simulink model "simulation"  (R2020b)
settings: Solver=VariableStepAuto  StartTime=0.0  StopTime=40  FixedStep=1e-3  RelTol=1e-3
values from neighbouring files (symbols this model uses):
  A0 = A- k*e1'    [script.m]
  ap = ssp.A'    [script.m]
  bp = ssp.C'    [script.m]
  c1 = 1    [script.m]
  c2 = 1    [script.m]
  cp = ssp.B'    [script.m]
  d1 = 1    [script.m]
  d2 = 1    [script.m]
  dp = 0    [script.m]
  e2 = [0 1]'    [script.m]
  gamma = 1    [script.m]
  Gamma = eye(3)    [script.m]
  k = 10*ones(n, 1)    [script.m]
  kp = 1    [script.m]
  rho0 = 0    [script.m]
  theta0 = zeros(3 , 1)    [script.m]
  x0p = zeros(n, 1)    [script.m]
settings Model: Creator=lucas  LastModifiedBy=lucas

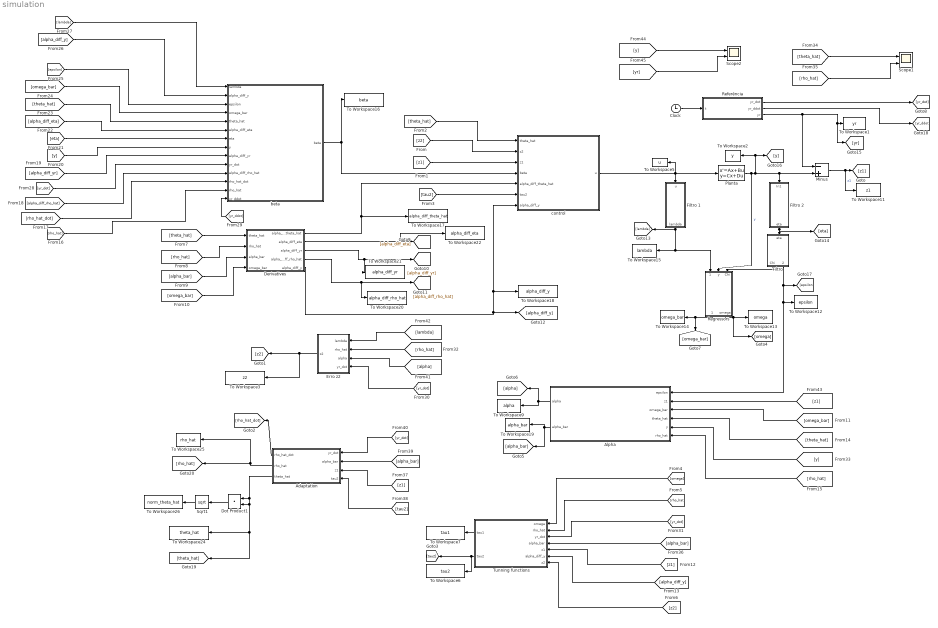
== system simulation ==
  Adaptation : Subsystem
  Alpha : MATLAB Function  TreatAsAtomicUnit=on
  Clock : Clock
  Derivatives : MATLAB Function  TreatAsAtomicUnit=on
  Dot Product1 : DotProduct  InputSameDT=on  OutDataTypeStr=Inherit: Inherit via internal rule
  Erro z2 : MATLAB Function  TreatAsAtomicUnit=on
  Filtro : MATLAB Function  TreatAsAtomicUnit=on
  Filtro 1 : Subsystem
  Filtro 2 : Subsystem
  Minus : Sum  Inputs=-+
  Planta : StateSpace  A=ap  B=bp  C=cp  D=dp  InitialCondition=x0p
  Referência : MATLAB Function  TreatAsAtomicUnit=on
  Regressors : MATLAB Function  TreatAsAtomicUnit=on
  Scope1 : Scope  NumInputPorts=2
  Scope2 : Scope  NumInputPorts=2
  Sqrt1 : Sqrt  SaturateOnIntegerOverflow=on
  To Workspace1 : ToWorkspace  VariableName=yr  SaveFormat=Timeseries  SampleTime=-1
  To Workspace11 : ToWorkspace  VariableName=z1  SaveFormat=Timeseries  SampleTime=-1
  To Workspace12 : ToWorkspace  VariableName=epsilon  SaveFormat=Timeseries  SampleTime=-1
  To Workspace13 : ToWorkspace  VariableName=omega  SaveFormat=Timeseries  SampleTime=-1
  To Workspace14 : ToWorkspace  VariableName=omega_bar  SaveFormat=Timeseries  SampleTime=-1
  To Workspace15 : ToWorkspace  VariableName=lambda  SaveFormat=Timeseries  SampleTime=-1
  To Workspace16 : ToWorkspace  VariableName=beta  SaveFormat=Timeseries  SampleTime=-1
  To Workspace17 : ToWorkspace  VariableName=alpha_diff_theta_hat  SaveFormat=Timeseries  SampleTime=-1
  To Workspace18 : ToWorkspace  VariableName=alpha_diff_y  SaveFormat=Timeseries  SampleTime=-1
  To Workspace19 : ToWorkspace  VariableName=alpha_bar  SaveFormat=Timeseries  SampleTime=-1
  To Workspace2 : ToWorkspace  VariableName=y  SaveFormat=Timeseries  SampleTime=-1
  To Workspace20 : ToWorkspace  VariableName=alpha_diff_rho_hat  SaveFormat=Timeseries  SampleTime=-1
  To Workspace21 : ToWorkspace  VariableName=alpha_diff_yr  SaveFormat=Timeseries  SampleTime=-1
  To Workspace22 : ToWorkspace  VariableName=alpha_diff_eta  SaveFormat=Timeseries  SampleTime=-1
  To Workspace24 : ToWorkspace  VariableName=theta_hat  SaveFormat=Timeseries  SampleTime=-1
  To Workspace25 : ToWorkspace  VariableName=rho_hat  SaveFormat=Timeseries  SampleTime=-1
  To Workspace26 : ToWorkspace  VariableName=norm_theta_hat  SaveFormat=Timeseries  SampleTime=-1
  To Workspace3 : ToWorkspace  VariableName=z2  SaveFormat=Timeseries  SampleTime=-1
  To Workspace5 : ToWorkspace  VariableName=u  SaveFormat=Timeseries  SampleTime=-1
  To Workspace6 : ToWorkspace  VariableName=tau2  SaveFormat=Timeseries  SampleTime=-1
  To Workspace7 : ToWorkspace  VariableName=tau1  SaveFormat=Timeseries  SampleTime=-1
  To Workspace9 : ToWorkspace  VariableName=alpha  SaveFormat=Timeseries  SampleTime=-1
  Tunning functions : MATLAB Function  TreatAsAtomicUnit=on
  beta : MATLAB Function  TreatAsAtomicUnit=on
  control : MATLAB Function  TreatAsAtomicUnit=on
  wires:
  [yr] -> Scope2/2
  [y] -> Scope2/1
  [alpha] -> Erro z2/3(alpha)
  Dot Product1/1 -> Sqrt1/1
  Sqrt1/1 -> To Workspace26/1
  [y] -> Alpha/5(y)
  Alpha/1(alpha) -> [alpha], To Workspace9/1
  [theta_hat] -> Alpha/4(theta_hat)
  [rho_hat] -> Alpha/6(rho_hat)
  Alpha/2(alpha_bar) -> To Workspace19/1, [alpha_bar]
  [z1] -> Alpha/2(z1)
  [omega_bar] -> beta/4(omega_bar)
  Derivatives/5(alpha_diff_y) -> control/7(alpha_diff_y), To Workspace18/1, [alpha_diff_y]
  Derivatives/1(alpha_diff_theta_hat) -> control/5(alpha_diff_theta_hat), To Workspace17/1
  [alpha_diff_y] -> beta/2(alpha_diff_y)
  [rho_hat] -> beta/13(rho_hat)
  [epsilon] -> beta/3(epsilon)
  [z2] -> control/2(z2)
  [lambda] -> beta/1(lambda)
  [alpha_diff_y] -> Tunning functions/6(alpha_diff_y)
  [theta_hat] -> beta/5(theta_hat)
  [eta] -> beta/7(eta)
  [omega_bar] -> Derivatives/4(omega_bar)
  [alpha_diff_yr] -> beta/9(alpha_diff_yr)
  [rho_hat] -> Tunning functions/2(rho_hat)
  [alpha_bar] -> Derivatives/3(alpha_bar)
  beta/1(beta) -> To Workspace16/1, control/4(beta)
  Derivatives/2(alpha_diff_eta) -> To Workspace22/1, [alpha_diff_eta]
  Regressors/1(omega_bar) -> To Workspace14/1, [omega_bar]
  Derivatives/4(alpha_diff_rho_hat) -> To Workspace20/1, [alpha_diff_rho_hat]
  Tunning functions/2(tau2) -> [tau2], To Workspace6/1
  [tau2] -> control/6(tau2)
  control/1(u) -> Filtro 1/1(u), To Workspace5/1, Planta/1
  [z1] -> control/3(z1)
  Filtro 1/1(lambda) -> Regressors/1(lambda), To Workspace15/1, [lambda]
  Planta/1 -> Minus/2, Filtro 2/1(In1), [y], To Workspace2/1, Regressors/2(y)  "y"
  Filtro 2/1(eta) -> Filtro/1(eta), [eta]
  Filtro/2(epsilon) -> Alpha/1(epsilon), To Workspace12/1, [epsilon]
  [alpha_diff_eta] -> beta/6(alpha_diff_eta)
  Referência/1(yr_dot) -> [yr_dot]
  [y] -> beta/8(y)
  [alpha_diff_rho_hat] -> beta/11(alpha_diff_rho_hat)
  Clock/1 -> Referência/1(t)
  Referência/2(yr_ddot) -> [yr_ddot]
  [theta_hat] -> Derivatives/1(theta_hat)
  Derivatives/3(alpha_diff_yr) -> To Workspace21/1, [alpha_diff_yr]
  [rho_hat_dot] -> beta/12(rho_hat_dot)
  [yr_ddot] -> beta/14(yr_ddot)
  [z2] -> Tunning functions/7(z2)
  [yr_dot] -> beta/10(yr_dot)
  [z1] -> Tunning functions/5(z1)
  [theta_hat] -> Scope1/1
  Tunning functions/1(tau1) -> To Workspace7/1
  [alpha_bar] -> Tunning functions/4(alpha_bar)
  [rho_hat] -> Scope1/2
  [rho_hat] -> Erro z2/2(rho_hat)
  Referência/3(yr) -> Minus/1, [yr], To Workspace1/1
  [omega_bar] -> Alpha/3(omega_bar)
  [rho_hat] -> Derivatives/2(rho_hat)
  [yr_dot] -> Erro z2/4(yr_dot)
  Minus/1 -> To Workspace11/1, [z1]  "z1"
  [lambda] -> Erro z2/1(lambda)
  [alpha_bar] -> Adaptation/2(alpha_bar)
  Adaptation/1(rho_hat_dot) -> [rho_hat_dot]
  [theta_hat] -> control/1(theta_hat)
  Adaptation/2(rho_hat) -> To Workspace25/1, [rho_hat]
  [omega] -> Tunning functions/1(omega)
  [yr_dot] -> Adaptation/1(yr_dot)
  [z1] -> Adaptation/3(z1)
  [yr_dot] -> Tunning functions/3(yr_dot)
  Adaptation/3(theta_hat) -> [theta_hat], To Workspace24/1, Dot Product1/2, Dot Product1/1
  [tau2] -> Adaptation/4(tau2)
  Regressors/2(omega) -> To Workspace13/1, [omega]
  Erro z2/1(z2) -> To Workspace3/1, [z2]
  Filtro/1(Chi) -> Regressors/3(Chi)

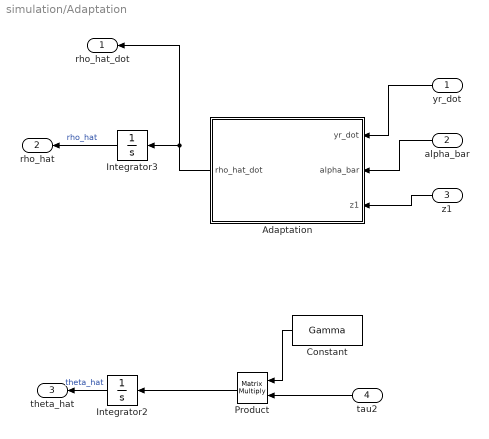
== system simulation/Adaptation ==
  yr_dot : Inport
  alpha_bar : Inport  Port=2
  z1 : Inport  Port=3
  tau2 : Inport  Port=4
  Adaptation : MATLAB Function  TreatAsAtomicUnit=on
  Constant : Constant  Value=Gamma  VectorParams1D=off
  Integrator2 : Integrator  InitialCondition=theta0
  Integrator3 : Integrator  InitialCondition=rho0
  Product : Product  Multiplication=Matrix(*)
  rho_hat_dot : Outport
  rho_hat : Outport  Port=2
  theta_hat : Outport  Port=3
  wires:
  Adaptation/1(rho_hat_dot) -> rho_hat_dot/1, Integrator3/1
  z1/1 -> Adaptation/3(z1)
  tau2/1 -> Product/2
  yr_dot/1 -> Adaptation/1(yr_dot)
  Constant/1 -> Product/1
  Product/1 -> Integrator2/1
  Integrator3/1 -> rho_hat/1  "rho_hat"
  alpha_bar/1 -> Adaptation/2(alpha_bar)
  Integrator2/1 -> theta_hat/1  "theta_hat"

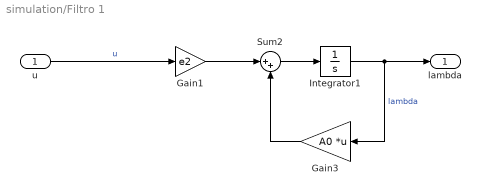
== system simulation/Filtro 1 ==
  u : Inport
  Gain1 : Gain  Gain=e2
  Gain3 : Gain  Gain=A0  Multiplication=Matrix(K*u) (u vector)
  Integrator1 : Integrator
  Sum2 : Sum  Inputs=|++
  lambda : Outport
  wires:
  u/1 -> Gain1/1  "u"
  Sum2/1 -> Integrator1/1
  Gain3/1 -> Sum2/2
  Gain1/1 -> Sum2/1
  Integrator1/1 -> lambda/1, Gain3/1  "lambda"

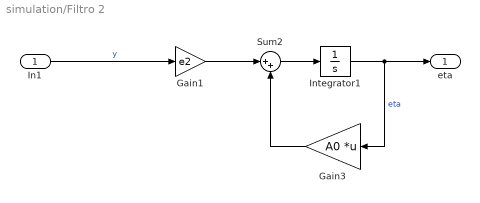
== system simulation/Filtro 2 ==
  In1 : Inport
  Gain1 : Gain  Gain=e2
  Gain3 : Gain  Gain=A0  Multiplication=Matrix(K*u) (u vector)
  Integrator1 : Integrator
  Sum2 : Sum  Inputs=|++
  eta : Outport
  wires:
  In1/1 -> Gain1/1  "y"
  Sum2/1 -> Integrator1/1
  Gain3/1 -> Sum2/2
  Gain1/1 -> Sum2/1
  Integrator1/1 -> eta/1, Gain3/1  "eta"

== matlab function simulation/control ==
  data: theta_hat input; u output; z2 input; z1 input; beta input; alpha_diff_theta_hat input; tau2 input; alpha_diff_y input; c2 parameter; d2 parameter; Gamma parameter
function u = control(theta_hat, z2, z1, beta, alpha_diff_theta_hat, tau2, alpha_diff_y, c2, d2, Gamma)
    kp_hat = theta_hat(1);
    u = -c2*z2;
    u = u - kp_hat*z1;
    u = u + beta;
    u = u + alpha_diff_theta_hat*Gamma*tau2;
    u = u - d2*(alpha_diff_y^2)*z2;

== matlab function simulation/Tunning functions ==
  data: omega input; tau1 output; rho_hat input; yr_dot input; alpha_bar input; z1 input; tau2 output; alpha_diff_y input; z2 input; e1_tau parameter
function [tau1, tau2] = tunning(omega, rho_hat, yr_dot, alpha_bar, z1, alpha_diff_y, z2, e1_tau)
    omega_0 = omega-(rho_hat*(yr_dot+alpha_bar)*e1_tau);
    tau1 = omega_0*z1;
    tau2 = tau1 - (alpha_diff_y*omega*z2);

== matlab function simulation/Referência ==
  data: yr_dot output; yr_ddot output; t input; yr output
function [yr_dot, yr_ddot, yr] = reference(t)
    yr = 2 + 5*sin(t) + 5*sin(3.7*t);
    yr_dot = 5*cos(t) + 5*3.7*cos(3.7*t);
    yr_ddot = -5*sin(t) - 5*3.7*3.7*sin(3.7*t);

== matlab function simulation/Erro z2 ==
  data: lambda input; z2 output; rho_hat input; alpha input; yr_dot input
function z2 = erro(lambda, rho_hat, alpha, yr_dot)
    z2 = lambda(2)-rho_hat*yr_dot - alpha;

== matlab function simulation/Adaptation/Adaptation ==
  data: yr_dot input; rho_hat_dot output; alpha_bar input; z1 input; gamma parameter; kp parameter
function rho_hat_dot  = adaptation(yr_dot, alpha_bar, z1, gamma, kp)
    rho_hat_dot = -gamma*sign(kp)*(yr_dot+alpha_bar)*z1;

== matlab function simulation/Alpha ==
  data: epsilon input; alpha output; z1 input; omega_bar input; theta_hat input; y input; rho_hat input; alpha_bar output; c1 parameter; d1 parameter
function [alpha, alpha_bar] = alpha(epsilon,z1, omega_bar, theta_hat, y, rho_hat, c1, d1)
    alpha_bar = -(c1*z1)-(d1*z1)-epsilon(2)-(dot(omega_bar, theta_hat));
    alpha = rho_hat*alpha_bar;

== matlab function simulation/Filtro ==
  data: Chi output; eta input; epsilon output; A0 parameter
function [Chi, epsilon] = filtro(eta, A0)
    Chi = -[A0*eta eta];
    epsilon = -A0*A0*eta;

== matlab function simulation/Regressors ==
  data: lambda input; y input; omega_bar output; omega output; Chi input; e1 parameter
function [omega_bar, omega] = fcn(lambda, y, Chi, e1)
aux = Chi(2,:) - y*e1';
omega_bar = [0 aux]';
omega = [lambda(2) aux]';

== matlab function simulation/Derivatives ==
  data: alpha_diff_theta_hat output; alpha_diff_eta output; alpha_diff_yr output; alpha_diff_rho_hat output; theta_hat input; alpha_diff_y output; rho_hat input; alpha_bar input; c1 parameter; d1 parameter; omega_bar input; e2 parameter; A0 parameter
function [alpha_diff_theta_hat, alpha_diff_eta, alpha_diff_yr, alpha_diff_rho_hat, alpha_diff_y] = derivate(theta_hat, rho_hat, alpha_bar, c1, d1, omega_bar, e2, A0)
    a1_hat = theta_hat(2);
    a0_hat = theta_hat(3);
    alpha_diff_y = rho_hat*(-c1-d1+a1_hat);
    A02 = A0^2;
    alpha_diff_eta = rho_hat*(A02(2,:) + a1_hat*A0(2,:) + a0_hat*e2');
    alpha_diff_yr = rho_hat*(c1+d1);
    alpha_diff_rho_hat = alpha_bar;
    alpha_diff_theta_hat = -rho_hat*(omega_bar');

== matlab function simulation/beta ==
  data: beta output; lambda input; alpha_diff_y input; epsilon input; omega_bar input; theta_hat input; alpha_diff_eta input; eta input; y input; alpha_diff_yr input; yr_dot input; alpha_diff_rho_hat input; rho_hat_dot input; rho_hat input; yr_ddot input; k parameter; e2 parameter; A0 parameter
function beta = beta(lambda, alpha_diff_y, epsilon, omega_bar, theta_hat, alpha_diff_eta, eta, y, alpha_diff_yr, yr_dot, alpha_diff_rho_hat, rho_hat_dot, rho_hat, yr_ddot, k, e2, A0)
    beta = k(2)*lambda(1);
    beta = beta + alpha_diff_y*(epsilon(2) + dot(omega_bar,theta_hat));
    beta = beta + alpha_diff_eta*(A0*eta + e2*y);
    beta = beta + alpha_diff_yr*yr_dot;
    beta = beta + rho_hat_dot*(yr_dot+alpha_diff_rho_hat);
    beta = beta + rho_hat*yr_ddot;
